simulink model "AutoRS_Blatt_und_Turm"  (R2022b)
settings: Solver=FixedStepAuto  StartTime=0.0  StopTime=50  FixedStep=1e-4  RelTol=1e-3
settings Model: Creator=Sebastian  LastModifiedBy=Sebastian

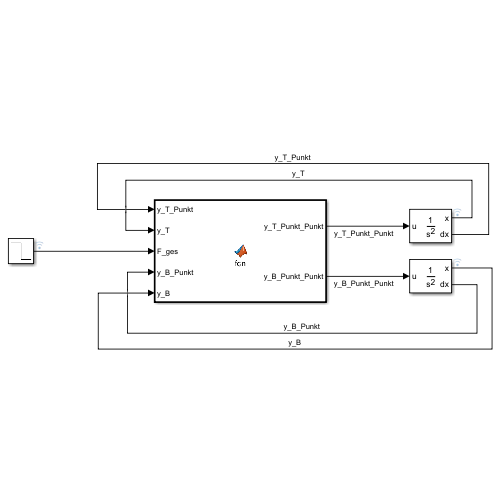
[thumbnail: Simulink's stored preview of the top-level diagram]
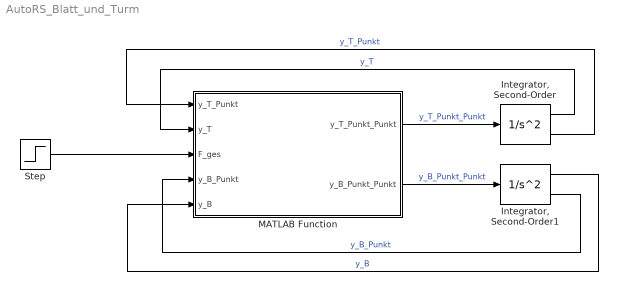
== system AutoRS_Blatt_und_Turm ==
  "Integrator, Second-Order" : SecondOrderIntegrator  ICX=0
  "Integrator, Second-Order1" : SecondOrderIntegrator  ICX=0
  MATLAB Function : MATLAB Function  TreatAsAtomicUnit=on
  Step : Step  Time=5  Before=(1/2)*1.225*63^2*pi*0.8*10  After=0  SampleTime=0
  wires:
  MATLAB Function/1(y_T_Punkt_Punkt) -> "Integrator, Second-Order"/1  "y_T_Punkt_Punkt"
  "Integrator, Second-Order"/2 -> MATLAB Function/1(y_T_Punkt)  "y_T_Punkt"
  "Integrator, Second-Order"/1 -> MATLAB Function/2(y_T)  "y_T"
  MATLAB Function/2(y_B_Punkt_Punkt) -> "Integrator, Second-Order1"/1  "y_B_Punkt_Punkt"
  "Integrator, Second-Order1"/2 -> MATLAB Function/4(y_B_Punkt)  "y_B_Punkt"
  "Integrator, Second-Order1"/1 -> MATLAB Function/5(y_B)  "y_B"
  Step/1 -> MATLAB Function/3(F_ges)

== matlab function AutoRS_Blatt_und_Turm/MATLAB Function ==
  data: y_T_Punkt input; y_T input; F_ges input; y_T_Punkt_Punkt output; y_B_Punkt input; y_B input; y_B_Punkt_Punkt output
function [y_T_Punkt_Punkt, y_B_Punkt_Punkt] = fcn(y_T_Punkt, y_T, F_ges, y_B_Punkt, y_B)

    % KONSTANTEN
    c = Konstanten();
    
    % BERECHNUNG
    y_T_Punkt_Punkt = (-c.k_T*y_T-c.d_T*y_T_Punkt+c.k_B*(y_B-y_T)+c.d_B*(y_B_Punkt-y_T_Punkt)+F_ges)/c.m_T;
    
    y_B_Punkt_Punkt = (-3*c.k_B*(y_B-y_T)-3*c.d_B*(y_B_Punkt-y_T_Punkt)+F_ges)/(3*c.m_B);

end
